simulink model "taque_simples"  (R2018b)
settings: Solver=VariableStepAuto  StartTime=0.0  StopTime=20  RelTol=1e-3
values from neighbouring files (symbols this model uses):
  A = double(subs(A,[h,u],[heq,ueq]))    [tanque_simples.m]
  B = double(subs(B,[h,u],[heq,ueq]))    [tanque_simples.m]
  heq = 1    [tanque_simples.m]
  ueq = double(solve(subs(f==0,h,heq),u))    [tanque_simples.m]
undefined symbols (not defined in the file or in its folder): uop
settings Model: Creator=bernardo  LastModifiedBy=bernardo

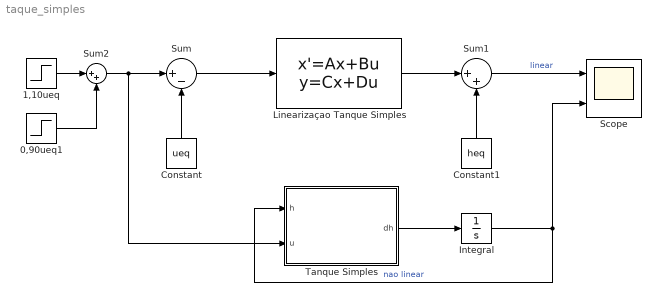
== system taque_simples ==
  0,90ueq1 : Step  Time=10  After=-0.2*uop  SampleTime=0
  1,10ueq : Step  Time=0  After=1.1*uop  SampleTime=0
  Constant : Constant  Value=ueq
  Constant1 : Constant  Value=heq
  Integral : Integrator  InitialCondition=1
  Linearizaçao Tanque Simples : StateSpace  A=A  B=B  D=0  InitialCondition=0
  Scope : Scope  NumInputPorts=2
  Sum : Sum  Inputs=|+-
  Sum1 : Sum  Inputs=|++
  Sum2 : Sum  Inputs=|++
  Tanque Simples : MATLAB Function  TreatAsAtomicUnit=on
  wires:
  Sum/1 -> Linearizaçao Tanque Simples/1
  Constant/1 -> Sum/2
  Linearizaçao Tanque Simples/1 -> Sum1/1
  Constant1/1 -> Sum1/2
  Sum1/1 -> Scope/1  "linear"
  Integral/1 -> Tanque Simples/1(h), Scope/2  "nao linear"
  Tanque Simples/1(dh) -> Integral/1
  1,10ueq/1 -> Sum2/1
  0,90ueq1/1 -> Sum2/2
  Sum2/1 -> Tanque Simples/2(u), Sum/1

== matlab function taque_simples/Tanque Simples ==
  data: h input; u input; dh output
function dh = fcn(h,u)
dh = 2.5*u - 0.6*sqrt(h);
end
